simulink model "DDCU_wxt_v03"  (R2014a)
settings: Solver=ode45  StartTime=0.0  StopTime=50  FixedStep=0.0005  RelTol=1e-3
values from neighbouring files (symbols this model uses):
  ag_thr = 0.4*g    (= 3.924)    [Veh_Par_wxt.m]
  B = 2.25    [Veh_Par_wxt.m]
  bra_pre_em = 12    [Veh_Par_wxt.m]
  bra_pre_gz2 = 12/3    (= 4)    [Veh_Par_wxt.m]
  bra_pre_gz34 = 12/3    (= 4)    [Veh_Par_wxt.m]
  bra_pre_yd = 12/2    (= 6)    [Veh_Par_wxt.m]
  brakepre_dem_data = [0 1 2 3 4 5 6 7 8 9 10 11 12]    [Veh_Par_wxt.m]
  brakeTrq_dem_data = [0 218.198 436.396 654.594 872.792 1090.99 1309.188 1527.386 1745.584 1963.782 2181.98 2400.178 2618.376]    [Veh_Par_wxt.m]
  bratrq_max = 4*2618.376    (= 10473.504)    [Veh_Par_wxt.m]
  eff_tran = 0.75    [Veh_Par_wxt.m]
  G = Mass*g    (= 36297)    [Veh_Par_wxt.m]
  kd1 = 1    [Veh_Par_wxt.m]
  kd2 = 1    [Veh_Par_wxt.m]
  kd3 = 1    [Veh_Par_wxt.m]
  ki1 = 1    [Veh_Par_wxt.m]
  ki2 = 1    [Veh_Par_wxt.m]
  ki3 = 1    [Veh_Par_wxt.m]
  kp1 = 1    [Veh_Par_wxt.m]
  kp2 = 1    [Veh_Par_wxt.m]
  kp3 = 1    [Veh_Par_wxt.m]
  L = 3.12    [Veh_Par_wxt.m]
  premax = 12    [Veh_Par_wxt.m]
  Radius = 0.20    (= 0.2)    [Veh_Par_wxt.m]
  s_opt_yi_add = 0.05    [Veh_Par_wxt.m]
  s_opt_zhuan_add = 0.05    [Veh_Par_wxt.m]
  spd_map_mot = [0 100 200 300 360 400 500 600 700 800 900]*tras_ratio    [Veh_Par_wxt.m]
  spdmax = 900*tras_ratio    (= 5580)    [Veh_Par_wxt.m]
  speed_thr_park = 5/3.6/Radius*30/pi    (= 66.3145596216)    [Veh_Par_wxt.m]
  tras_ratio = 6.2    [Veh_Par_wxt.m]
  trq_map_mot = [1200 1200 1200 1200 1200 1080 864 720 617 540 480]/tras_ratio    [Veh_Par_wxt.m]
  trqmax = 80    [Veh_Par_wxt.m]
  v_thr1_b = 5    [Veh_Par_wxt.m]
  v_thr2_b = 20    [Veh_Par_wxt.m]
  v_thr_park = 5    [Veh_Par_wxt.m]
undefined symbols (not defined in the file or in its folder): DiscIntNeverNeededParam
libraries: simulink x34, Solver_SF x1
(part 4 of 10)

== system DDCU_wxt_v03/MainControl/mode_control/center_steer/center_steer/左右侧电机分配及功率限制 ==
  steer_dem : Inport
  pwr_dis_bat : Inport  Port=2
  speed_act_lf : Inport  Port=3
  speed_act_lr : Inport  Port=4
  speed_act_rf : Inport  Port=5
  speed_act_rr : Inport  Port=6
  TrqLimU_dig_lf : Inport  Port=7
  TrqLimU_dig_lr : Inport  Port=8
  TrqLimU_dig_rf : Inport  Port=9
  TrqLimU_dig_rr : Inport  Port=10
  Abs : Abs
  Add1 : Sum  Inputs=++++
  Add3 : Sum  Inputs=++++
  Constant : Constant  Value=9549
  Divide : Product  Inputs=**/
  Gain : Gain  Gain=1/4
  Gain1 : Gain  Gain=1/2
  Gain2 : Gain  Gain=1/100
  MinMax{,3..6} (5 alike) : MinMax  Inputs=2
  Product : Product
  mot_map{,1..3} (4 alike) : Lookup_n-D  NumberOfTableDimensions=1  BreakpointsForDimension1=spd_map_mot  Table=trq_map_mot  InternalRulePriority=Speed  RndMeth=Simplest  InputSameDT=on
  trq_dem_l : Outport
  trq_dem_r : Outport  Port=2
  trqlim_lf : Outport  Port=3
  trqlim_lr : Outport  Port=4
  trqlim_rf : Outport  Port=5
  trqlim_rr : Outport  Port=6
  wires:
  speed_act_rf/1 -> mot_map2/1, Add1/3
  speed_act_lr/1 -> mot_map1/1, Add1/2
  speed_act_rr/1 -> mot_map3/1, Add1/4
  speed_act_lf/1 -> mot_map/1, Add1/1
  Add1/1 -> Gain/1
  Constant/1 -> Divide/1
  pwr_dis_bat/1 -> Divide/2
  Gain/1 -> Divide/3
  mot_map3/1 -> MinMax3/1
  TrqLimU_dig_rr/1 -> MinMax3/2
  mot_map2/1 -> MinMax4/1
  TrqLimU_dig_rf/1 -> MinMax4/2
  mot_map1/1 -> MinMax5/1
  TrqLimU_dig_lr/1 -> MinMax5/2
  mot_map/1 -> MinMax6/1
  TrqLimU_dig_lf/1 -> MinMax6/2
  MinMax6/1 -> trqlim_lf/1, Add3/1
  MinMax5/1 -> trqlim_lr/1, Add3/2
  MinMax4/1 -> trqlim_rf/1, Add3/3
  MinMax3/1 -> trqlim_rr/1, Add3/4
  Divide/1 -> MinMax/1
  Add3/1 -> MinMax/2
  MinMax/1 -> Product/2
  steer_dem/1 -> Abs/1
  Product/1 -> Gain1/1
  Gain1/1 -> trq_dem_r/1, trq_dem_l/1
  Gain2/1 -> Product/1
  Abs/1 -> Gain2/1

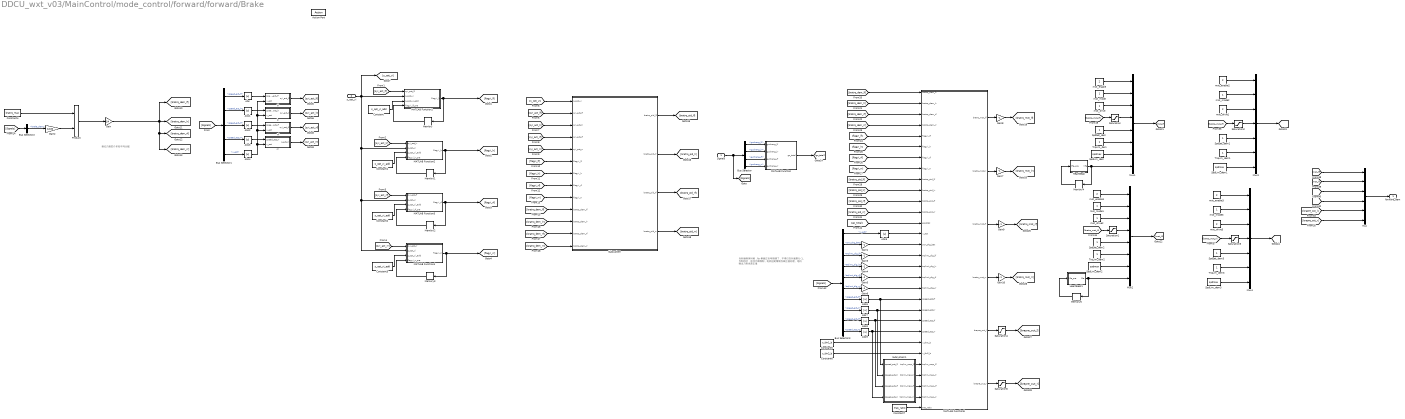
== system DDCU_wxt_v03/MainControl/mode_control/forward/forward/Brake ==
  note: 当时编程序时候，fcn里面正负号搞错了，不得已在外面乘以-1，
      | 当制动时，电池功率限制，电机扭矩限制当做正值处理，电机
      | 输出力矩也是正值
  note: 制动力矩四个车轮平均分配
  Signals : Inport
  s_opt_yi : Inport  Port=2
  Action Port : ActionPort
  Abs{,1..9} (10 alike) : Abs
  Bus Selector : BusSelector  OutputSignals=DriveMotor.guzhang_lf,DriveMotor.guzhang_lr,DriveMotor.guzhang_rf,DriveMotor.guzhang_rr
  Bus Selector1 : BusSelector  OutputSignals=DriveMotor.speed_act_lf,DriveMotor.speed_act_lr,DriveMotor.speed_act_rf,DriveMotor.speed_act_rr,IMU.v_act
  Bus Selector2 : BusSelector  OutputSignals=YaoKong.brake_dem
  Bus Selector3 : BusSelector  OutputSignals=IMU.v_act,Bat.pwr_chg_bat,DriveMotor.trqlimL_dig_lf,DriveMotor.trqlimL_dig_lr,DriveMotor.trqlimL_dig_rf,DriveMotor.trqlimL_dig_rr,DriveMotor.speed_act_lf,DriveMotor.speed_act_lr,DriveMotor.speed_act_rf,DriveMotor.speed_act_rr
  Constant{,1..3} (4 alike) : Constant  Value=s_opt_yi_add
  Constant4 : Constant  Value=bratrq_max
  Constant5 : Constant  Value=v_thr1_b
  Constant6 : Constant  Value=v_thr2_b
  Constant7 : Constant  Value=tras_ratio
  Gain : Gain  Gain=1/4
  Gain{1,3..10} (9 alike) : Gain  Gain=-1
  Gain2 : Gain  Gain=1/100
  HeartBeat : MATLAB Function  TreatAsAtomicUnit=on
  HeartBeat1 : MATLAB Function  TreatAsAtomicUnit=on
  MATLAB Function : MATLAB Function  TreatAsAtomicUnit=on
  MATLAB Function1 : MATLAB Function  TreatAsAtomicUnit=on
  MATLAB Function2 : MATLAB Function  TreatAsAtomicUnit=on
  MATLAB Function3 : MATLAB Function  TreatAsAtomicUnit=on
  MATLAB Function4 : MATLAB Function  TreatAsAtomicUnit=on
  MATLAB Function5 : MATLAB Function  TreatAsAtomicUnit=on
  Memory{,1..5} (6 alike) : Memory  InheritSampleTime=on
  Mux : Mux  Inputs=6
  Mux1 : Mux  Inputs=8
  Mux2 : Mux  Inputs=8
  Mux3 : Mux  Inputs=7
  Mux4 : Mux  Inputs=7
  Product : Product
  Saturation{,1..3} (4 alike) : Saturate  UpperLimit=0  LowerLimit=-trqmax
  Saturation4 : Saturate  UpperLimit=premax  LowerLimit=0
  Saturation5 : Saturate  UpperLimit=premax  LowerLimit=0
  SpdLim_dem{,1..3} (4 alike) : Constant  Value=spdmax
  SpdSet_dem{,1..3} (4 alike) : Constant
  Subsystem : Subsystem
  Subsystem1 : Subsystem
  TrqLim_dem{,1..3} (4 alike) : Constant
  lf : Subsystem
  lr : Subsystem
  mot_drive : Constant
  mot_drive1 : Constant  Value=2
  mot_drive2 : Constant
  mot_drive3 : Constant  Value=2
  mot_enable{,1..3} (4 alike) : Constant  Value=2
  mot_mode{,1..3} (4 alike) : Constant
  rf : Subsystem
  rr : Subsystem
  forward_dem : Outport
  wires:
  Signals/1 -> [Signals], Bus Selector/1
  Bus Selector/3 -> MATLAB Function/3(guzhang_rf)  "<guzhang_rf>"
  Bus Selector/4 -> MATLAB Function/4(guzhang_rr)  "<guzhang_rr>"
  Bus Selector/2 -> MATLAB Function/2(guzhang_lr)  "<guzhang_lr>"
  Bus Selector/1 -> MATLAB Function/1(guzhang_lf)  "<guzhang_lf>"
  MATLAB Function/1(gz_total) -> [gz_total]
  [Signals] -> Bus Selector1/1
  Bus Selector1/1 -> Abs/1  "<speed_act_lf>"
  Bus Selector1/2 -> Abs1/1  "<speed_act_lr>"
  Bus Selector1/3 -> Abs2/1  "<speed_act_rf>"
  Bus Selector1/4 -> Abs3/1  "<speed_act_rr>"
  Bus Selector1/5 -> Abs4/1  "<v_act>"
  Constant3/1 -> MATLAB Function4/3(s_opt_yi_add)
  Memory3/1 -> MATLAB Function4/4(flagyi_rr_pre)
  MATLAB Function4/1(flagyi_rr) -> Memory3/1, [flagyi_rr]
  s_opt_yi/1 -> MATLAB Function2/2(s_opt_yi), MATLAB Function3/2(s_opt_yi), MATLAB Function4/2(s_opt_yi), MATLAB Function1/2(s_opt_yi), [s_opt_yi]
  Constant2/1 -> MATLAB Function3/3(s_opt_yi_add)
  Memory2/1 -> MATLAB Function3/4(flagyi_rf_pre)
  MATLAB Function3/1(flagyi_rf) -> [flagyi_rf], Memory2/1
  Constant1/1 -> MATLAB Function2/3(s_opt_yi_add)
  Memory1/1 -> MATLAB Function2/4(flagyi_lr_pre)
  MATLAB Function2/1(flagyi_lr) -> Memory1/1, [flagyi_lr]
  Constant/1 -> MATLAB Function1/3(s_opt_yi_add)
  Memory/1 -> MATLAB Function1/4(flagyi_lf_pre)
  MATLAB Function1/1(flagyi_lf) -> [flagyi_lf], Memory/1
  lr/1(syi_act_lr) -> [syi_act_lr]
  lf/1(syi_act_lf) -> [syi_act_lf]
  rf/1(syi_act_rf) -> [syi_act_rf]
  rr/1(s_act_rr) -> [syi_act_rr]
  [syi_act_lf] -> MATLAB Function1/1(syi_act_lf)
  [syi_act_lr] -> MATLAB Function2/1(syi_act_lr)
  [syi_act_rf] -> MATLAB Function3/1(syi_act_rf)
  [syi_act_rr] -> MATLAB Function4/1(syi_act_rr)
  [s_opt_yi] -> Subsystem/1(s_opt_yi)
  [syi_act_lf] -> Subsystem/2(syi_act_lf)
  [syi_act_lr] -> Subsystem/3(syi_act_lr)
  [syi_act_rf] -> Subsystem/4(syi_act_rf)
  [syi_act_rr] -> Subsystem/5(syi_act_rr)
  [flagyi_rf] -> Subsystem/8(flagyi_rf)
  [flagyi_lf] -> Subsystem/6(flagyi_lf)
  [flagyi_lr] -> Subsystem/7(flagyi_lr)
  [flagyi_rr] -> Subsystem/9(flagyi_rr)
  [Signals] -> Bus Selector2/1
  Gain/1 -> [bratrq_dem_lr], [bratrq_dem_rr], [bratrq_dem_rf], [bratrq_dem_lf]
  [bratrq_dem_lf] -> Subsystem/10(bratrq_dem_lf)
  [bratrq_dem_lr] -> Subsystem/11(bratrq_dem_lr)
  [bratrq_dem_rf] -> Subsystem/12(bratrq_dem_rf)
  [bratrq_dem_rr] -> Subsystem/13(bratrq_dem_rr)
  Subsystem/2(bratrq_pid_lr) -> [bratrq_pid_lr]
  Subsystem/3(bratrq_pid_rf) -> [bratrq_pid_rf]
  Subsystem/1(bratrq_pid_lf) -> [bratrq_pid_lf]
  Subsystem/4(bratrq_pid_rr) -> [bratrq_pid_rr]
  Mux/1 -> forward_dem/1
  SpdLim_dem3/1 -> Mux4/7
  TrqLim_dem3/1 -> Mux4/6
  Mux4/1 -> [mot_rr]
  SpdSet_dem3/1 -> Mux4/5
  mot_enable3/1 -> Mux4/1
  [bratrq_mot_rr] -> Saturation3/1
  mot_mode3/1 -> Mux4/2
  mot_drive3/1 -> Mux4/3
  SpdLim_dem2/1 -> Mux2/7
  Memory5/1 -> HeartBeat1/1(life_pre)
  HeartBeat1/1(life) -> Memory5/1, Mux2/8
  TrqLim_dem2/1 -> Mux2/6
  Mux2/1 -> [mot_lr]
  SpdSet_dem2/1 -> Mux2/5
  mot_enable1/1 -> Mux2/1
  [bratrq_mot_lr] -> Saturation1/1
  mot_mode1/1 -> Mux2/2
  mot_drive2/1 -> Mux2/3
  SpdLim_dem1/1 -> Mux3/7
  TrqLim_dem1/1 -> Mux3/6
  Mux3/1 -> [mot_rf]
  SpdSet_dem1/1 -> Mux3/5
  mot_enable2/1 -> Mux3/1
  [bratrq_mot_rf] -> Saturation2/1
  mot_mode2/1 -> Mux3/2
  mot_drive1/1 -> Mux3/3
  SpdLim_dem/1 -> Mux1/7
  Memory4/1 -> HeartBeat/1(life_pre)
  HeartBeat/1(life) -> Memory4/1, Mux1/8
  TrqLim_dem/1 -> Mux1/6
  Mux1/1 -> [mot_lf]
  SpdSet_dem/1 -> Mux1/5
  mot_enable/1 -> Mux1/1
  mot_mode/1 -> Mux1/2
  mot_drive/1 -> Mux1/3
  [mot_lf] -> Mux/1
  [mot_lr] -> Mux/2
  [mot_rf] -> Mux/3
  [mot_rr] -> Mux/4
  [brapre_out_l] -> Mux/5
  [brapre_out_r] -> Mux/6
  MATLAB Function5/1(bratrq_mot_lf) -> Gain8/1
  MATLAB Function5/3(bratrq_mot_rf) -> Gain9/1
  MATLAB Function5/2(bratrq_mot_lr) -> Gain7/1
  MATLAB Function5/4(bratrq_mot_rr) -> Gain10/1
  MATLAB Function5/5(brapre_out_l) -> Saturation4/1
  MATLAB Function5/6(brapre_out_r) -> Saturation5/1
  [Signals] -> Bus Selector3/1
  Bus Selector3/2 -> Gain1/1  "<pwr_chg_bat>"
  Bus Selector3/1 -> Abs5/1  "<v_act>"
  Bus Selector3/3 -> Gain3/1  "<trqlimL_dig_lf>"
  Bus Selector3/4 -> Gain4/1  "<trqlimL_dig_lr>"
  Bus Selector3/5 -> Gain5/1  "<trqlimL_dig_rf>"
  Bus Selector3/6 -> Gain6/1  "<trqlimL_dig_rr>"
  Bus Selector3/7 -> Abs6/1  "<speed_act_lf>"
  Bus Selector3/8 -> Abs7/1  "<speed_act_lr>"
  Bus Selector3/9 -> Abs8/1  "<speed_act_rf>"
  Bus Selector3/10 -> Abs9/1  "<speed_act_rr>"
  Constant4/1 -> Product/1
  Gain2/1 -> Product/2
  Bus Selector2/1 -> Gain2/1  "<brake_dem>"
  Product/1 -> Gain/1
  Constant6/1 -> MATLAB Function5/25(v_thr2_b)
  Gain1/1 -> MATLAB Function5/15(pwr_chg_bat)
  Gain3/1 -> MATLAB Function5/16(trqlimL_dig_lf)
  Gain4/1 -> MATLAB Function5/17(trqlimL_dig_lr)
  Gain5/1 -> MATLAB Function5/18(trqlimL_dig_rf)
  Gain6/1 -> MATLAB Function5/19(trqlimL_dig_rr)
  [bratrq_dem_lr] -> MATLAB Function5/2(bratrq_dem_lr)
  [bratrq_dem_rf] -> MATLAB Function5/3(bratrq_dem_rf)
  [bratrq_dem_lf] -> MATLAB Function5/1(bratrq_dem_lf)
  [bratrq_dem_rr] -> MATLAB Function5/4(bratrq_dem_rr)
  [flagyi_lf] -> MATLAB Function5/5(flagyi_lf)
  [flagyi_lr] -> MATLAB Function5/6(flagyi_lr)
  [flagyi_rf] -> MATLAB Function5/7(flagyi_rf)
  [flagyi_rr] -> MATLAB Function5/8(flagyi_rr)
  [bratrq_pid_lf] -> MATLAB Function5/9(bratrq_pid_lf)
  [bratrq_pid_lr] -> MATLAB Function5/10(bratrq_pid_lr)
  [bratrq_pid_rf] -> MATLAB Function5/11(bratrq_pid_rf)
  [bratrq_pid_rr] -> MATLAB Function5/12(bratrq_pid_rr)
  [gz_total] -> MATLAB Function5/13(gz_total)
  Subsystem1/4(trqlim_map_rr) -> MATLAB Function5/29(trqlim_map_rr)
  Subsystem1/3(trqlim_map_rf) -> MATLAB Function5/28(trqlim_map_rf)
  Subsystem1/2(trqlim_map_lr) -> MATLAB Function5/27(trqlim_map_lr)
  Subsystem1/1(trqlim_map_lf) -> MATLAB Function5/26(trqlim_map_lf)
  Constant5/1 -> MATLAB Function5/24(v_thr1_b)
  [bratrq_mot_lf] -> Saturation/1
  Gain8/1 -> [bratrq_mot_lf]
  Gain7/1 -> [bratrq_mot_lr]
  Gain9/1 -> [bratrq_mot_rf]
  Gain10/1 -> [bratrq_mot_rr]
  Saturation/1 -> Mux1/4
  Saturation1/1 -> Mux2/4
  Saturation2/1 -> Mux3/4
  Saturation3/1 -> Mux4/4
  Saturation4/1 -> [brapre_out_l]
  Saturation5/1 -> [brapre_out_r]
  Abs/1 -> lf/1(speed_act_lf)
  Abs1/1 -> lr/1(speed_act_lr)
  Abs2/1 -> rf/1(speed_act_rf)
  Abs3/1 -> rr/1(speed_act_rr)
  Abs4/1 -> rr/2(v_act), rf/2(v_act), lr/2(v_act), lf/2(v_act)
  Abs5/1 -> MATLAB Function5/14(v_act)
  Abs6/1 -> Subsystem1/1(speed_act_lf), MATLAB Function5/20(speed_act_lf)
  Abs7/1 -> Subsystem1/2(speed_act_lr), MATLAB Function5/21(speed_act_lr)
  Abs8/1 -> Subsystem1/3(speed_act_rf), MATLAB Function5/22(speed_act_rf)
  Abs9/1 -> Subsystem1/4(speed_act_rr), MATLAB Function5/23(speed_act_rr)
  Constant7/1 -> MATLAB Function5/30(tras_ratio)

== system DDCU_wxt_v03/MainControl/mode_control/forward/forward/Drive ==
  Signals : Inport
  Action Port : ActionPort
  Abs{,1..10} (11 alike) : Abs
  Bus Selector : BusSelector  OutputSignals=YaoKong.acc_dem,IMU.v_act,DriveMotor.trqlimU_dig_lf,DriveMotor.trqlimU_dig_lr,DriveMotor.trqlimU_dig_rf,DriveMotor.trqlimU_dig_rr
  Bus Selector1 : BusSelector  OutputSignals=IMU.acc_y
  Bus Selector2 : BusSelector  OutputSignals=IMU.acc_y,YaoKong.steer_dem
  Bus Selector3 : BusSelector  OutputSignals=IMU.dis_east,IMU.dis_north,IMU.hangxiangangle
  Bus Selector4 : BusSelector  OutputSignals=IMU.v_act,DriveMotor.trqlimU_dig_lf,DriveMotor.trqlimU_dig_lr,DriveMotor.trqlimU_dig_rf,DriveMotor.trqlimU_dig_rr,YaoKong.steer_dem
  Bus Selector5 : BusSelector  OutputSignals=Bat.pwr_dis_bat,DriveMotor.speed_act_lf,DriveMotor.speed_act_lr,DriveMotor.speed_act_rf,DriveMotor.speed_act_rr,DriveMotor.trqlimU_dig_lf,DriveMotor.trqlimU_dig_lr,DriveMotor.trqlimU_dig_rf,DriveMotor.trqlimU_dig_rr
  Bus Selector6 : BusSelector  OutputSignals=DriveMotor.guzhang_lf,DriveMotor.guzhang_lr,DriveMotor.guzhang_rf,DriveMotor.guzhang_rr
  Bus Selector7 : BusSelector  OutputSignals=DriveMotor.speed_act_lf,DriveMotor.speed_act_lr,DriveMotor.speed_act_rf,DriveMotor.speed_act_rr,IMU.v_act,YaoKong.steer_dem,IMU.acc_y,YaoKong.brake_dem
  Constant : Constant  Value=ag_thr
  Constant1 : Constant
  MATLAB Function : MATLAB Function  TreatAsAtomicUnit=on
  Multiport Switch : MultiPortSwitch  DataPortOrder=Zero-based contiguous
  Scope : Scope
      settings: SaveName=ScopeData5
  Scope1 : Scope
      settings: SaveName=ScopeData6
  Scope2 : Scope
      settings: SaveName=ScopeData9
  Switch Case : SwitchCase  CaseConditions={0,1,2}  ShowDefaultCase=off
  Terminator : Terminator
  容错控制 : Subsystem
  左右侧电机分配及功率限制 : Subsystem
  目标直驶力矩确定模块 : Subsystem
  目标转向力矩确定模块 : Subsystem  TreatAsAtomicUnit=on
  直驶纠偏控制 : Subsystem  TreatAsAtomicUnit=on
  路面状况识别模块 : Subsystem
  车辆稳定性控制 : Subsystem  TreatAsAtomicUnit=on
  驱动防滑控制TCS : Subsystem
  forward_dem : Outport
  wires:
  Signals/1 -> [Signals], Bus Selector4/1, Bus Selector3/1, Bus Selector1/1, Bus Selector2/1, Bus Selector/1
  Bus Selector/1 -> 目标直驶力矩确定模块/1(acc_dem)  "<acc_dem>"
  Bus Selector/2 -> Abs9/1  "<v_act>"
  Bus Selector1/1 -> 车辆稳定性控制/1(acc_y)  "<acc_y>"
  MATLAB Function/1(y) -> Scope2/1, Multiport Switch/1, Switch Case/1
  Switch Case/1 -> 车辆稳定性控制/Action
  Switch Case/2 -> 目标转向力矩确定模块/Action
  Switch Case/3 -> 直驶纠偏控制/Action
  车辆稳定性控制/1(delta_Twending_dem) -> Multiport Switch/2
  目标转向力矩确定模块/1(delta_Tsteer_dem) -> Scope/1, Multiport Switch/3
  直驶纠偏控制/1(delta_Tjiupian) -> Multiport Switch/4
  Bus Selector2/2 -> MATLAB Function/2(steer_dem)  "<steer_dem>"
  Constant/1 -> MATLAB Function/3(ag_thr)
  [umax] -> 目标转向力矩确定模块/7(umax)
  [f] -> 目标转向力矩确定模块/8(f)
  路面状况识别模块/1(umax) -> [umax]
  路面状况识别模块/2(f) -> [f]
  路面状况识别模块/3(s_opt_zhuan) -> [s_opt_zhuan]
  Bus Selector3/1 -> 直驶纠偏控制/1(dis_east)  "<dis_east>"
  Bus Selector3/2 -> 直驶纠偏控制/2(dis_north)  "<dis_north>"
  Bus Selector3/3 -> 直驶纠偏控制/3(hangxiangangle)  "<hangxiangangle>"
  Multiport Switch/1 -> Scope1/1, 左右侧电机分配及功率限制/2(delta_T_dem)
  目标直驶力矩确定模块/1(Trq_line_dem) -> 左右侧电机分配及功率限制/1(Trq_line_dem)
  Bus Selector/4 -> 目标直驶力矩确定模块/4(TrqLimU_dig_lr)  "<trqlimU_dig_lr>"
  Bus Selector/3 -> 目标直驶力矩确定模块/3(TrqLimU_dig_lf)  "<trqlimU_dig_lf>"
  Bus Selector/5 -> 目标直驶力矩确定模块/5(TrqLimU_dig_rf)  "<trqlimU_dig_rf>"
  Bus Selector/6 -> 目标直驶力矩确定模块/6(TrqLimU_dig_rr)  "<trqlimU_dig_rr>"
  Bus Selector4/4 -> 目标转向力矩确定模块/4(TrqLimU_dig_rf)  "<trqlimU_dig_rf>"
  Bus Selector4/5 -> 目标转向力矩确定模块/5(TrqLimU_dig_rr)  "<trqlimU_dig_rr>"
  Bus Selector4/6 -> 目标转向力矩确定模块/6(steer_dem)  "<steer_dem>"
  Bus Selector4/1 -> Abs10/1  "<v_act>"
  Bus Selector4/2 -> 目标转向力矩确定模块/2(TrqLimU_dig_lf)  "<trqlimU_dig_lf>"
  Bus Selector4/3 -> 目标转向力矩确定模块/3(TrqLimU_dig_lr)  "<trqlimU_dig_lr>"
  Bus Selector2/1 -> MATLAB Function/1(acc_y)  "<acc_y>"
  [Signals] -> Bus Selector5/1
  Bus Selector5/1 -> 左右侧电机分配及功率限制/3(pwr_dis_bat)  "<pwr_dis_bat>"
  Bus Selector5/2 -> Abs/1  "<speed_act_lf>"
  Bus Selector5/3 -> Abs1/1  "<speed_act_lr>"
  Bus Selector5/4 -> Abs2/1  "<speed_act_rf>"
  Bus Selector5/5 -> Abs3/1  "<speed_act_rr>"
  Bus Selector5/9 -> 左右侧电机分配及功率限制/11(TrqLimU_dig_rr)  "<trqlimU_dig_rr>"
  Bus Selector5/8 -> 左右侧电机分配及功率限制/10(TrqLimU_dig_rf)  "<trqlimU_dig_rf>"
  Bus Selector5/6 -> 左右侧电机分配及功率限制/8(TrqLimU_dig_lf)  "<trqlimU_dig_lf>"
  Bus Selector5/7 -> 左右侧电机分配及功率限制/9(TrqLimU_dig_lr)  "<trqlimU_dig_lr>"
  [Signals] -> Bus Selector6/1
  左右侧电机分配及功率限制/2(trq_dem_r) -> 容错控制/2(trq_dem_r)
  左右侧电机分配及功率限制/1(trq_dem_l) -> 容错控制/1(trq_dem_l)
  Bus Selector6/4 -> 容错控制/10(guzhang_rr)  "<guzhang_rr>"
  Bus Selector6/3 -> 容错控制/9(guzhang_rf)  "<guzhang_rf>"
  Bus Selector6/2 -> 容错控制/8(guzhang_lr)  "<guzhang_lr>"
  Bus Selector6/1 -> 容错控制/7(guzhang_lf)  "<guzhang_lf>"
  左右侧电机分配及功率限制/5(trqlim_rf) -> 容错控制/5(trqlim_rf)
  左右侧电机分配及功率限制/4(trqlim_lr) -> 容错控制/4(trqlim_lr)
  左右侧电机分配及功率限制/6(trqlim_rr) -> 容错控制/6(trqlim_rr)
  左右侧电机分配及功率限制/3(trqlim_lf) -> 容错控制/3(trqlim_lf)
  容错控制/1(trq_dem_lf) -> 驱动防滑控制TCS/1(trq_dem_lf)
  容错控制/5(bra_pre_l) -> 驱动防滑控制TCS/5(bra_pre_l)
  容错控制/6(bra_pre_r) -> 驱动防滑控制TCS/6(bra_pre_r)
  容错控制/2(trq_dem_lr) -> 驱动防滑控制TCS/2(trq_dem_lr)
  容错控制/3(trq_dem_rf) -> 驱动防滑控制TCS/3(trq_dem_rf)
  容错控制/4(trq_dem_rr) -> 驱动防滑控制TCS/4(trq_dem_rr)
  Bus Selector7/7 -> 驱动防滑控制TCS/13(acc_y)  "<acc_y>"
  Bus Selector7/6 -> 驱动防滑控制TCS/12(steer_dem)  "<steer_dem>"
  Bus Selector7/5 -> Abs8/1  "<v_act>"
  Bus Selector7/4 -> Abs7/1  "<speed_act_rr>"
  Bus Selector7/3 -> Abs6/1  "<speed_act_rf>"
  Bus Selector7/2 -> Abs5/1  "<speed_act_lr>"
  Bus Selector7/1 -> Abs4/1  "<speed_act_lf>"
  [s_opt_zhuan] -> 驱动防滑控制TCS/15(s_opt_zhuan)
  Bus Selector7/8 -> 驱动防滑控制TCS/14(brake_dem)  "<brake_dem>"
  [Signals] -> Bus Selector7/1
  驱动防滑控制TCS/1(forward_dem) -> forward_dem/1
  Constant1/1 -> 路面状况识别模块/1(In1)
  路面状况识别模块/4(s_opt_yi) -> Terminator/1
  Abs/1 -> 左右侧电机分配及功率限制/4(speed_act_lf)
  Abs1/1 -> 左右侧电机分配及功率限制/5(speed_act_lr)
  Abs2/1 -> 左右侧电机分配及功率限制/6(speed_act_rf)
  Abs3/1 -> 左右侧电机分配及功率限制/7(speed_act_rr)
  Abs4/1 -> 驱动防滑控制TCS/7(speed_act_lf)
  Abs5/1 -> 驱动防滑控制TCS/8(speed_act_lr)
  Abs6/1 -> 驱动防滑控制TCS/9(speed_act_rf)
  Abs7/1 -> 驱动防滑控制TCS/10(speed_act_rr)
  Abs8/1 -> 驱动防滑控制TCS/11(v_act)
  Abs9/1 -> 目标直驶力矩确定模块/2(v_act)
  Abs10/1 -> 目标转向力矩确定模块/1(v_act)

== system DDCU_wxt_v03/MainControl/mode_control/backward/backward/Brake/Subsystem ==
  s_opt_yi : Inport
  syi_act_lf : Inport  Port=2
  syi_act_lr : Inport  Port=3
  syi_act_rf : Inport  Port=4
  syi_act_rr : Inport  Port=5
  flagyi_lf : Inport  Port=6
  flagyi_lr : Inport  Port=7
  flagyi_rf : Inport  Port=8
  flagyi_rr : Inport  Port=9
  bratrq_dem_lf : Inport  Port=10
  bratrq_dem_lr : Inport  Port=11
  bratrq_dem_rf : Inport  Port=12
  bratrq_dem_rr : Inport  Port=13
  Add{1..2,5,7} (4 alike) : Sum  Inputs=+++
  Add{3..4,6,8} (4 alike) : Sum
  Difference{,1..3} (4 alike) : simulink/Discrete/Difference  ICPrevInput=0.0  InputProcessing=Inherited  OutMin=[]  OutMax=[]  OutDataType=fixdt(1, 16)  OutScaling=2^-10  DoSatur=off
  Discrete-Time Integrator{,1..3} (4 alike) : DiscreteIntegrator  SampleTime=-1  ICPrevOutput=DiscIntNeverNeededParam  ICPrevScaledInput=DiscIntNeverNeededParam
  Gain{1,4,7,10} (4 alike) : Gain  Gain=kp3
  Gain{2,5,8,11} (4 alike) : Gain  Gain=ki3
  Gain{3,6,9,12} (4 alike) : Gain  Gain=kd3
  Sum{,1..3} (4 alike) : Sum  Inputs=|+-
  Switch{,1..3} (4 alike) : Switch  Criteria=u2 > Threshold  Threshold=0.5
  bratrq_pid_lf : Outport
  bratrq_pid_lr : Outport  Port=2
  bratrq_pid_rf : Outport  Port=3
  bratrq_pid_rr : Outport  Port=4
  wires:
  Sum2/1 -> Gain7/1, Gain9/1, Gain8/1
  Add5/1 -> Add6/1
  Sum3/1 -> Gain10/1, Gain12/1, Gain11/1
  Add7/1 -> Add8/1
  Sum1/1 -> Gain4/1, Gain5/1, Gain6/1
  Sum/1 -> Gain1/1, Gain3/1, Gain2/1
  Switch3/1 -> bratrq_pid_rf/1
  flagyi_rf/1 -> Switch3/2
  [s_opt_yi] -> Sum3/1
  Gain11/1 -> Discrete-Time Integrator3/1
  Gain10/1 -> Add7/1
  Gain12/1 -> Difference3/1
  Discrete-Time Integrator3/1 -> Add7/2
  Difference3/1 -> Add7/3
  syi_act_rf/1 -> Sum3/2
  bratrq_dem_rf/1 -> Add8/2, Switch3/3
  Add8/1 -> Switch3/1
  Switch2/1 -> bratrq_pid_rr/1
  flagyi_rr/1 -> Switch2/2
  [s_opt_yi] -> Sum2/1
  Gain8/1 -> Discrete-Time Integrator2/1
  Gain7/1 -> Add5/1
  Gain9/1 -> Difference2/1
  Discrete-Time Integrator2/1 -> Add5/2
  Difference2/1 -> Add5/3
  syi_act_rr/1 -> Sum2/2
  bratrq_dem_rr/1 -> Add6/2, Switch2/3
  Add6/1 -> Switch2/1
  Switch1/1 -> bratrq_pid_lr/1
  flagyi_lr/1 -> Switch1/2
  [s_opt_yi] -> Sum1/1
  Gain5/1 -> Discrete-Time Integrator1/1
  Gain4/1 -> Add1/1
  Gain6/1 -> Difference1/1
  Discrete-Time Integrator1/1 -> Add1/2
  Difference1/1 -> Add1/3
  syi_act_lr/1 -> Sum1/2
  bratrq_dem_lr/1 -> Add4/2, Switch1/3
  Add4/1 -> Switch1/1
  Switch/1 -> bratrq_pid_lf/1
  flagyi_lf/1 -> Switch/2
  s_opt_yi/1 -> Sum/1, [s_opt_yi]
  Gain2/1 -> Discrete-Time Integrator/1
  Gain1/1 -> Add2/1
  Gain3/1 -> Difference/1
  Discrete-Time Integrator/1 -> Add2/2
  Difference/1 -> Add2/3
  syi_act_lf/1 -> Sum/2
  bratrq_dem_lf/1 -> Add3/2, Switch/3
  Add3/1 -> Switch/1
  Add2/1 -> Add3/1
  Add1/1 -> Add4/1

== system DDCU_wxt_v03/MainControl/mode_control/backward/backward/Brake/Subsystem1 ==
  speed_act_lf : Inport
  speed_act_lr : Inport  Port=2
  speed_act_rf : Inport  Port=3
  speed_act_rr : Inport  Port=4
  mot_map{,1..3} (4 alike) : Lookup_n-D  NumberOfTableDimensions=1  BreakpointsForDimension1=spd_map_mot  Table=trq_map_mot  InternalRulePriority=Speed  RndMeth=Simplest  InputSameDT=on
  trqlim_map_lf : Outport
  trqlim_map_lr : Outport  Port=2
  trqlim_map_rf : Outport  Port=3
  trqlim_map_rr : Outport  Port=4
  wires:
  mot_map3/1 -> trqlim_map_rr/1
  mot_map2/1 -> trqlim_map_rf/1
  mot_map1/1 -> trqlim_map_lr/1
  mot_map/1 -> trqlim_map_lf/1
  speed_act_rr/1 -> mot_map3/1
  speed_act_rf/1 -> mot_map2/1
  speed_act_lr/1 -> mot_map1/1
  speed_act_lf/1 -> mot_map/1

== system DDCU_wxt_v03/MainControl/mode_control/backward/backward/Brake/lf ==
  speed_act_lf : Inport
  v_act : Inport  Port=2
  Add : Sum
  Constant : Constant  Value=eps
  Divide : Product  Inputs=*/
  Gain : Gain  Gain=pi/30
  Gain1 : Gain  Gain=Radius
  Gain2 : Gain  Gain=1/3.6
  Subtract : Sum  Inputs=+-
  syi_act_lf : Outport
  wires:
  Gain1/1 -> Subtract/2
  Gain2/1 -> Subtract/1, Add/1
  speed_act_lf/1 -> Gain/1
  Gain/1 -> Gain1/1
  v_act/1 -> Gain2/1
  Subtract/1 -> Divide/1
  Constant/1 -> Add/2
  Add/1 -> Divide/2
  Divide/1 -> syi_act_lf/1

== system DDCU_wxt_v03/MainControl/mode_control/backward/backward/Brake/lr ==
  speed_act_lr : Inport
  v_act : Inport  Port=2
  Add : Sum
  Constant : Constant  Value=eps
  Divide : Product  Inputs=*/
  Gain : Gain  Gain=pi/30
  Gain1 : Gain  Gain=Radius
  Gain2 : Gain  Gain=1/3.6
  Subtract : Sum  Inputs=+-
  syi_act_lr : Outport
  wires:
  Gain2/1 -> Subtract/1, Add/1
  Gain1/1 -> Subtract/2
  Divide/1 -> syi_act_lr/1
  Add/1 -> Divide/2
  Constant/1 -> Add/2
  Subtract/1 -> Divide/1
  v_act/1 -> Gain2/1
  Gain/1 -> Gain1/1
  speed_act_lr/1 -> Gain/1

== system DDCU_wxt_v03/MainControl/mode_control/backward/backward/Brake/rf ==
  speed_act_rf : Inport
  v_act : Inport  Port=2
  Add : Sum
  Constant : Constant  Value=eps
  Divide : Product  Inputs=*/
  Gain : Gain  Gain=pi/30
  Gain1 : Gain  Gain=Radius
  Gain2 : Gain  Gain=1/3.6
  Subtract : Sum  Inputs=+-
  syi_act_rf : Outport
  wires:
  Gain1/1 -> Subtract/2
  Gain2/1 -> Subtract/1, Add/1
  speed_act_rf/1 -> Gain/1
  Gain/1 -> Gain1/1
  v_act/1 -> Gain2/1
  Subtract/1 -> Divide/1
  Constant/1 -> Add/2
  Add/1 -> Divide/2
  Divide/1 -> syi_act_rf/1

== system DDCU_wxt_v03/MainControl/mode_control/backward/backward/Brake/rr ==
  speed_act_rr : Inport
  v_act : Inport  Port=2
  Add : Sum
  Constant : Constant  Value=eps
  Divide : Product  Inputs=*/
  Gain : Gain  Gain=pi/30
  Gain1 : Gain  Gain=Radius
  Gain2 : Gain  Gain=1/3.6
  Subtract : Sum  Inputs=+-
  s_act_rr : Outport
  wires:
  Gain1/1 -> Subtract/2
  Gain2/1 -> Subtract/1, Add/1
  Divide/1 -> s_act_rr/1
  Add/1 -> Divide/2
  Constant/1 -> Add/2
  Subtract/1 -> Divide/1
  v_act/1 -> Gain2/1
  Gain/1 -> Gain1/1
  speed_act_rr/1 -> Gain/1

== system DDCU_wxt_v03/MainControl/mode_control/backward/backward/Drive/容错控制 ==
  trq_dem_l : Inport
  trq_dem_r : Inport  Port=2
  trqlim_lf : Inport  Port=3
  trqlim_lr : Inport  Port=4
  trqlim_rf : Inport  Port=5
  trqlim_rr : Inport  Port=6
  guzhang_lf : Inport  Port=7
  guzhang_lr : Inport  Port=8
  guzhang_rf : Inport  Port=9
  guzhang_rr : Inport  Port=10
  Add : Sum
  Add1 : Sum
  Constant : Constant  Value=bra_pre_gz2
  Constant1 : Constant  Value=bra_pre_gz34
  MATLAB Function : MATLAB Function  TreatAsAtomicUnit=on
  Mux : Mux  Inputs=2
  Scope{,1..16} (17 alike) : Scope
      Scope settings: SaveName=ScopeData25
      Scope1 settings: SaveName=ScopeData26
      Scope10 settings: SaveName=ScopeData35
      Scope11 settings: SaveName=ScopeData36
      Scope12 settings: SaveName=ScopeData37
      Scope13 settings: SaveName=ScopeData38
      Scope14 settings: SaveName=ScopeData39
      Scope15 settings: SaveName=ScopeData40
      Scope16 settings: SaveName=ScopeData41
      Scope2 settings: SaveName=ScopeData27
      Scope3 settings: SaveName=ScopeData28
      Scope4 settings: SaveName=ScopeData29
      Scope5 settings: SaveName=ScopeData30
      Scope6 settings: SaveName=ScopeData31
      Scope7 settings: SaveName=ScopeData32
      Scope8 settings: SaveName=ScopeData33
      Scope9 settings: SaveName=ScopeData34
  Subtract : Sum  Inputs=+-
  trq_dem_lf : Outport
  trq_dem_lr : Outport  Port=2
  trq_dem_rf : Outport  Port=3
  trq_dem_rr : Outport  Port=4
  bra_pre_l : Outport  Port=5
  bra_pre_r : Outport  Port=6
  wires:
  MATLAB Function/7(mode) -> Scope11/1
  Mux/1 -> Scope7/1
  Subtract/1 -> Scope6/1
  Add1/1 -> Subtract/2, Mux/2
  Add/1 -> Subtract/1, Mux/1
  Constant1/1 -> MATLAB Function/12(bra_pre_gz34)
  Constant/1 -> MATLAB Function/11(bra_pre_gz2)
  MATLAB Function/6(bra_pre_r) -> bra_pre_r/1, Scope5/1
  MATLAB Function/5(bra_pre_l) -> bra_pre_l/1, Scope4/1
  MATLAB Function/4(trq_dem_rr) -> trq_dem_rr/1, Add1/2, Scope3/1
  MATLAB Function/3(trq_dem_rf) -> trq_dem_rf/1, Add1/1, Scope2/1
  MATLAB Function/2(trq_dem_lr) -> trq_dem_lr/1, Add/2, Scope1/1
  MATLAB Function/1(trq_dem_lf) -> trq_dem_lf/1, Add/1, Scope/1
  trqlim_lf/1 -> MATLAB Function/3(trqlim_lf)
  trqlim_rr/1 -> MATLAB Function/6(trqlim_rr), Scope12/1
  trqlim_rf/1 -> MATLAB Function/5(trqlim_rf), Scope10/1
  trq_dem_l/1 -> MATLAB Function/1(trq_dem_l), Scope8/1
  trqlim_lr/1 -> MATLAB Function/4(trqlim_lr)
  trq_dem_r/1 -> MATLAB Function/2(trq_dem_r), Scope9/1
  guzhang_lf/1 -> MATLAB Function/7(guzhang_lf), Scope13/1
  guzhang_rr/1 -> MATLAB Function/10(guzhang_rr), Scope16/1
  guzhang_rf/1 -> MATLAB Function/9(guzhang_rf), Scope15/1
  guzhang_lr/1 -> Scope14/1, MATLAB Function/8(guzhang_lr)

== system DDCU_wxt_v03/MainControl/mode_control/backward/backward/Drive/左右侧电机分配及功率限制 ==
  Trq_line_dem : Inport
  delta_T_dem : Inport  Port=2
  pwr_dis_bat : Inport  Port=3
  speed_act_lf : Inport  Port=4
  speed_act_lr : Inport  Port=5
  speed_act_rf : Inport  Port=6
  speed_act_rr : Inport  Port=7
  TrqLimU_dig_lf : Inport  Port=8
  TrqLimU_dig_lr : Inport  Port=9
  TrqLimU_dig_rf : Inport  Port=10
  TrqLimU_dig_rr : Inport  Port=11
  Add : Sum
  Add1 : Sum  Inputs=++++
  Add2 : Sum
  Add3 : Sum
  Constant : Constant  Value=9549
  Divide : Product  Inputs=**/
  Gain : Gain  Gain=1/4
  Gain1 : Gain  Gain=1/2
  Gain2 : Gain  Gain=1/2
  MATLAB Function : MATLAB Function  TreatAsAtomicUnit=on
  MinMax{,1..6} (7 alike) : MinMax  Inputs=2
  Mux : Mux  Inputs=2
  Scope{,1..10} (11 alike) : Scope
      Scope settings: SaveName=ScopeData14
      Scope1 settings: SaveName=ScopeData15
      Scope10 settings: SaveName=ScopeData24
      Scope2 settings: SaveName=ScopeData16
      Scope3 settings: SaveName=ScopeData17
      Scope4 settings: SaveName=ScopeData18
      Scope5 settings: SaveName=ScopeData19
      Scope6 settings: SaveName=ScopeData20
      Scope7 settings: SaveName=ScopeData21
      Scope8 settings: SaveName=ScopeData22
      Scope9 settings: SaveName=ScopeData23
  Subtract : Sum  Inputs=+-
  mot_map{,1..3} (4 alike) : Lookup_n-D  NumberOfTableDimensions=1  BreakpointsForDimension1=spd_map_mot  Table=trq_map_mot  InternalRulePriority=Speed  RndMeth=Simplest  InputSameDT=on
  trq_dem_l : Outport
  trq_dem_r : Outport  Port=2
  trqlim_lf : Outport  Port=3
  trqlim_lr : Outport  Port=4
  trqlim_rf : Outport  Port=5
  trqlim_rr : Outport  Port=6
  wires:
  Gain2/1 -> Mux/2, Subtract/2, Add/2, Scope6/1
  Mux/1 -> Scope5/1
  MATLAB Function/2(trq_dem_r) -> trq_dem_r/1, Scope1/1
  MATLAB Function/1(trq_dem_l) -> trq_dem_l/1, Scope/1
  [delta_T_dem] -> MATLAB Function/5(delta_T_dem)
  [trqlim_r] -> Scope9/1, MinMax2/1, MATLAB Function/3(trqlim_r)
  Add2/1 -> [trqlim_r]
  [trqlim_l] -> MinMax1/1, MATLAB Function/1(trqlim_l), Scope4/1
  Add3/1 -> [trqlim_l]
  MinMax3/1 -> Add2/2, trqlim_rr/1
  MinMax4/1 -> Add2/1, trqlim_rf/1
  MinMax5/1 -> Add3/2, trqlim_lr/1
  MinMax6/1 -> Add3/1, trqlim_lf/1
  TrqLimU_dig_lf/1 -> MinMax6/2
  mot_map/1 -> MinMax6/1
  TrqLimU_dig_lr/1 -> MinMax5/2
  mot_map1/1 -> MinMax5/1
  TrqLimU_dig_rf/1 -> MinMax4/2
  mot_map2/1 -> MinMax4/1
  TrqLimU_dig_rr/1 -> MinMax3/2
  mot_map3/1 -> MinMax3/1
  MinMax2/1 -> MATLAB Function/4(trq_dem_r1), Scope7/1
  Add/1 -> MinMax2/2, Scope8/1
  MinMax1/1 -> MATLAB Function/2(trq_dem_l1), Scope3/1
  Subtract/1 -> MinMax1/2, Scope2/1
  delta_T_dem/1 -> Gain2/1, Scope10/1, [delta_T_dem]
  Gain1/1 -> Add/1, Subtract/1, Mux/1
  MinMax/1 -> Gain1/1
  Trq_line_dem/1 -> MinMax/2
  Divide/1 -> MinMax/1
  Gain/1 -> Divide/3
  pwr_dis_bat/1 -> Divide/2
  Constant/1 -> Divide/1
  Add1/1 -> Gain/1
  speed_act_lf/1 -> Add1/1, mot_map/1
  speed_act_rr/1 -> Add1/4, mot_map3/1
  speed_act_lr/1 -> Add1/2, mot_map1/1
  speed_act_rf/1 -> Add1/3, mot_map2/1

== system DDCU_wxt_v03/MainControl/mode_control/backward/backward/Drive/目标直驶力矩确定模块 ==
  acc_dem : Inport
  v_act : Inport  Port=2
  TrqLimU_dig_lf : Inport  Port=3
  TrqLimU_dig_lr : Inport  Port=4
  TrqLimU_dig_rf : Inport  Port=5
  TrqLimU_dig_rr : Inport  Port=6
  Add : Sum  Inputs=++++
  Constant : Constant  Value=3.6
  Constant1 : Constant  Value=Radius
  Constant2 : Constant  Value=30/pi
  Divide : Product  Inputs=*//*
  Gain : Gain  Gain=1/100
  Gain1 : Gain  Gain=tras_ratio
  MinMax{,1..3} (4 alike) : MinMax  Inputs=2
  Product : Product
  Scope : Scope
      settings: SaveName=ScopeData7
  Scope1 : Scope
      settings: SaveName=ScopeData8
  mot_map : Lookup_n-D  NumberOfTableDimensions=1  BreakpointsForDimension1=spd_map_mot  Table=trq_map_mot  InternalRulePriority=Speed  RndMeth=Simplest  InputSameDT=on
  Trq_line_dem : Outport
  wires:
  Gain1/1 -> mot_map/1
  Gain/1 -> Product/1
  Product/1 -> Trq_line_dem/1, Scope/1
  acc_dem/1 -> Gain/1
  Add/1 -> Product/2
  MinMax3/1 -> Add/4
  MinMax/1 -> Add/1
  MinMax2/1 -> Add/3
  MinMax1/1 -> Add/2
  TrqLimU_dig_rr/1 -> MinMax3/2
  TrqLimU_dig_rf/1 -> MinMax2/2
  TrqLimU_dig_lr/1 -> MinMax1/2
  mot_map/1 -> MinMax/1, Scope1/1, MinMax3/1, MinMax2/1, MinMax1/1
  TrqLimU_dig_lf/1 -> MinMax/2
  Divide/1 -> Gain1/1
  Constant2/1 -> Divide/4
  Constant/1 -> Divide/2
  Constant1/1 -> Divide/3
  v_act/1 -> Divide/1

== system DDCU_wxt_v03/MainControl/mode_control/backward/backward/Drive/目标转向力矩确定模块 ==
  note: 左转为正，右转为负
  v_act : Inport
  TrqLimU_dig_lf : Inport  Port=2
  TrqLimU_dig_lr : Inport  Port=3
  TrqLimU_dig_rf : Inport  Port=4
  TrqLimU_dig_rr : Inport  Port=5
  steer_dem : Inport  Port=6
  umax : Inport  Port=7
  f : Inport  Port=8
  Action Port : ActionPort
  Add : Sum
  Add1 : Sum
  Constant : Constant  Value=3.6
  Constant1 : Constant  Value=Radius
  Constant2 : Constant  Value=30/pi
  Constant3 : Constant  Value=G
  Constant4 : Constant  Value=L
  Constant5 : Constant  Value=B
  Constant6 : Constant  Value=eff_tran
  Constant7 : Constant  Value=Radius
  Constant8 : Constant  Value=ag_thr
  Constant9 : Constant  Value=Radius
  Divide : Product  Inputs=*//*
  Gain : Gain  Gain=1/100
  Gain1 : Gain  Gain=tras_ratio
  Gain2 : Gain  Gain=tras_ratio
  Gain3 : Gain  Gain=tras_ratio
  Gain4 : Gain  Gain=1/tras_ratio
  MATLAB Function : MATLAB Function  TreatAsAtomicUnit=on
  MATLAB Function1 : MATLAB Function  TreatAsAtomicUnit=on
  MATLAB Function2 : MATLAB Function  TreatAsAtomicUnit=on
  MinMax{,1..3} (4 alike) : MinMax  Inputs=2
  MinMax4 : MinMax  Function=max  Inputs=2
  Product : Product
  Scope{,1..3} (4 alike) : Scope
      Scope settings: SaveName=ScopeData10
      Scope1 settings: SaveName=ScopeData11
      Scope2 settings: SaveName=ScopeData12
      Scope3 settings: SaveName=ScopeData13
  mot_map : Lookup_n-D  NumberOfTableDimensions=1  BreakpointsForDimension1=spd_map_mot  Table=trq_map_mot  InternalRulePriority=Speed  RndMeth=Simplest  InputSameDT=on
  delta_Tsteer_dem : Outport
  wires:
  Gain1/1 -> mot_map/1
  MATLAB Function2/1(delta_Tsteer_max) -> Product/2, Scope2/1
  MinMax4/1 -> MATLAB Function2/6(Rturn_min_xy)
  Constant9/1 -> MATLAB Function2/5(Radius)
  [B] -> MATLAB Function2/4(B)
  [L] -> MATLAB Function2/3(L)
  [G] -> MATLAB Function2/2(G)
  [umax] -> MATLAB Function2/1(umax)
  MATLAB Function1/1(Rturn_min_ag) -> Scope1/1, MinMax4/2
  Constant8/1 -> MATLAB Function1/2(ag_thr)
  [v_act] -> MATLAB Function1/1(v_act)
  MATLAB Function/1(Rturn_min) -> MinMax4/1, Scope/1
  f/1 -> MATLAB Function/10(f)
  Constant7/1 -> MATLAB Function/9(Radius)
  Constant6/1 -> MATLAB Function/8(eff_tran)
  Add1/1 -> Gain3/1
  Add/1 -> Gain2/1
  umax/1 -> MATLAB Function/4(umax), [umax]
  Constant5/1 -> MATLAB Function/5(B), [B]
  Constant4/1 -> MATLAB Function/3(L), [L]
  Constant3/1 -> MATLAB Function/2(G), [G]
  steer_dem/1 -> MATLAB Function/1(steer_dem), [steer_dem]
  v_act/1 -> Divide/1, [v_act]
  Constant1/1 -> Divide/3
  Constant/1 -> Divide/2
  Constant2/1 -> Divide/4
  Divide/1 -> Gain1/1
  TrqLimU_dig_lf/1 -> MinMax/2
  mot_map/1 -> MinMax1/1, MinMax2/1, MinMax3/1, MinMax/1
  TrqLimU_dig_lr/1 -> MinMax1/2
  TrqLimU_dig_rf/1 -> MinMax2/2
  TrqLimU_dig_rr/1 -> MinMax3/2
  MinMax1/1 -> Add/2
  MinMax2/1 -> Add1/1
  MinMax/1 -> Add/1
  MinMax3/1 -> Add1/2
  [steer_dem] -> Gain/1
  Product/1 -> Gain4/1, Scope3/1
  Gain/1 -> Product/1
  Gain2/1 -> MATLAB Function/6(Tpeak_L)
  Gain3/1 -> MATLAB Function/7(Tpeak_R)
  Gain4/1 -> delta_Tsteer_dem/1

== system DDCU_wxt_v03/MainControl/mode_control/backward/backward/Drive/直驶纠偏控制 ==
  dis_east : Inport
  dis_north : Inport  Port=2
  hangxiangangle : Inport  Port=3
  Action Port : ActionPort
  Constant : Constant  Value=0
  Terminator : Terminator
  Terminator1 : Terminator
  Terminator2 : Terminator
  delta_Tjiupian : Outport
  wires:
  hangxiangangle/1 -> Terminator2/1
  dis_north/1 -> Terminator1/1
  dis_east/1 -> Terminator/1
  Constant/1 -> delta_Tjiupian/1

== system DDCU_wxt_v03/MainControl/mode_control/backward/backward/Drive/路面状况识别模块 ==
  In1 : Inport
  Constant : Constant  Value=0.9
  Constant1 : Constant  Value=0.05
  Constant2 : Constant  Value=0.15
  Constant3 : Constant  Value=0.15
  Terminator : Terminator
  umax : Outport
  f : Outport  Port=2
  s_opt_zhuan : Outport  Port=3
  s_opt_yi : Outport  Port=4
  wires:
  In1/1 -> Terminator/1
  Constant3/1 -> s_opt_yi/1
  Constant2/1 -> s_opt_zhuan/1
  Constant1/1 -> f/1
  Constant/1 -> umax/1

== system DDCU_wxt_v03/MainControl/mode_control/backward/backward/Drive/车辆稳定性控制 ==
  note: 加速度向左为正
  acc_y : Inport
  Action Port : ActionPort
  Abs : Abs
  Add : Sum  Inputs=+++
  Constant : Constant  Value=ag_thr
  Constant1 : Constant
  Constant2 : Constant  Value=-1
  Difference : simulink/Discrete/Difference  ICPrevInput=0.0  InputProcessing=Inherited  OutMin=[]  OutMax=[]  OutDataType=fixdt(1, 16)  OutScaling=2^-10  DoSatur=off
  Discrete-Time Integrator : DiscreteIntegrator  SampleTime=-1  ICPrevOutput=DiscIntNeverNeededParam  ICPrevScaledInput=DiscIntNeverNeededParam
  Gain : Gain  Gain=kp1
  Gain1 : Gain  Gain=ki1
  Gain2 : Gain  Gain=kd1
  Gain3 : Gain  Gain=1/tras_ratio
  Product : Product
  Sum : Sum  Inputs=|+-
  Switch : Switch
  delta_Twending_dem : Outport
  wires:
  Difference/1 -> Add/3
  Discrete-Time Integrator/1 -> Add/2
  Sum/1 -> Gain/1, Gain1/1, Gain2/1
  Add/1 -> Product/1
  Product/1 -> Gain3/1
  Switch/1 -> Product/2
  Constant2/1 -> Switch/3
  Constant1/1 -> Switch/1
  Abs/1 -> Sum/2
  Gain2/1 -> Difference/1
  Gain1/1 -> Discrete-Time Integrator/1
  Gain/1 -> Add/1
  acc_y/1 -> Abs/1, Switch/2
  Constant/1 -> Sum/1
  Gain3/1 -> delta_Twending_dem/1

== system DDCU_wxt_v03/MainControl/mode_control/backward/backward/Drive/驱动防滑控制TCS ==
  trq_dem_lf : Inport
  trq_dem_lr : Inport  Port=2
  trq_dem_rf : Inport  Port=3
  trq_dem_rr : Inport  Port=4
  bra_pre_l : Inport  Port=5
  bra_pre_r : Inport  Port=6
  speed_act_lf : Inport  Port=7
  speed_act_lr : Inport  Port=8
  speed_act_rf : Inport  Port=9
  speed_act_rr : Inport  Port=10
  v_act : Inport  Port=11
  steer_dem : Inport  Port=12
  acc_y : Inport  Port=13
  brake_dem : Inport  Port=14
  s_opt_zhuan : Inport  Port=15
  MATLAB Function : MATLAB Function  TreatAsAtomicUnit=on
  Multiport Switch : MultiPortSwitch  DataPortOrder=Zero-based contiguous  Inputs=2
  Switch Case : SwitchCase  CaseConditions={0,1}  ShowDefaultCase=off
  直行TCS : Subsystem  TreatAsAtomicUnit=on
  转向TCS : Subsystem  TreatAsAtomicUnit=on
  backward_dem : Outport
  wires:
  Multiport Switch/1 -> backward_dem/1
  转向TCS/1(backward_dem) -> Multiport Switch/2
  直行TCS/1(backward_dem) -> Multiport Switch/3
  brake_dem/1 -> 转向TCS/14(brake_dem), 直行TCS/14(brake_dem)
  s_opt_zhuan/1 -> 转向TCS/15(s_opt_zhuan), 直行TCS/15(s_opt_zhuan)
  acc_y/1 -> 转向TCS/13(acc_y), 直行TCS/13(acc_y)
  v_act/1 -> 转向TCS/12(v_act), 直行TCS/12(v_act)
  speed_act_rr/1 -> 转向TCS/11(speed_act_rr), 直行TCS/11(speed_act_rr)
  speed_act_rf/1 -> 转向TCS/10(speed_act_rf), 直行TCS/10(speed_act_rf)
  speed_act_lr/1 -> 转向TCS/9(speed_act_lr), 直行TCS/9(speed_act_lr)
  speed_act_lf/1 -> 转向TCS/8(speed_act_lf), 直行TCS/8(speed_act_lf)
  bra_pre_r/1 -> 转向TCS/7(bra_pre_r), 直行TCS/7(bra_pre_r)
  bra_pre_l/1 -> 转向TCS/6(bra_pre_l), 直行TCS/6(bra_pre_l)
  trq_dem_rr/1 -> 转向TCS/5(trq_dem_rr), 直行TCS/5(trq_dem_rr)
  trq_dem_rf/1 -> 转向TCS/4(trq_dem_rf), 直行TCS/4(trq_dem_rf)
  trq_dem_lr/1 -> 转向TCS/3(trq_dem_lr), 直行TCS/3(trq_dem_lr)
  trq_dem_lf/1 -> 转向TCS/2(trq_dem_lf), 直行TCS/2(trq_dem_lf)
  Switch Case/2 -> 直行TCS/Action
  Switch Case/1 -> 转向TCS/Action
  MATLAB Function/1(y) -> Switch Case/1, Multiport Switch/1
  steer_dem/1 -> MATLAB Function/1(steer_dem), 直行TCS/1(steer_dem), 转向TCS/1(steer_dem)

== system DDCU_wxt_v03/MainControl/mode_control/forward/forward/Brake/Subsystem ==
  s_opt_yi : Inport
  syi_act_lf : Inport  Port=2
  syi_act_lr : Inport  Port=3
  syi_act_rf : Inport  Port=4
  syi_act_rr : Inport  Port=5
  flagyi_lf : Inport  Port=6
  flagyi_lr : Inport  Port=7
  flagyi_rf : Inport  Port=8
  flagyi_rr : Inport  Port=9
  bratrq_dem_lf : Inport  Port=10
  bratrq_dem_lr : Inport  Port=11
  bratrq_dem_rf : Inport  Port=12
  bratrq_dem_rr : Inport  Port=13
  Add{1..2,5,7} (4 alike) : Sum  Inputs=+++
  Add{3..4,6,8} (4 alike) : Sum
  Difference{,1..3} (4 alike) : simulink/Discrete/Difference  ICPrevInput=0.0  InputProcessing=Inherited  OutMin=[]  OutMax=[]  OutDataType=fixdt(1, 16)  OutScaling=2^-10  DoSatur=off
  Discrete-Time Integrator{,1..3} (4 alike) : DiscreteIntegrator  SampleTime=-1  ICPrevOutput=DiscIntNeverNeededParam  ICPrevScaledInput=DiscIntNeverNeededParam
  Gain{1,4,7,10} (4 alike) : Gain  Gain=kp3
  Gain{2,5,8,11} (4 alike) : Gain  Gain=ki3
  Gain{3,6,9,12} (4 alike) : Gain  Gain=kd3
  Sum{,1..3} (4 alike) : Sum  Inputs=|+-
  Switch{,1..3} (4 alike) : Switch  Criteria=u2 > Threshold  Threshold=0.5
  bratrq_pid_lf : Outport
  bratrq_pid_lr : Outport  Port=2
  bratrq_pid_rf : Outport  Port=3
  bratrq_pid_rr : Outport  Port=4
  wires:
  Add3/1 -> Switch/1
  bratrq_dem_lf/1 -> Switch/3, Add3/2
  syi_act_lf/1 -> Sum/2
  Difference/1 -> Add2/3
  Discrete-Time Integrator/1 -> Add2/2
  Gain3/1 -> Difference/1
  Gain1/1 -> Add2/1
  Gain2/1 -> Discrete-Time Integrator/1
  s_opt_yi/1 -> [s_opt_yi], Sum/1
  flagyi_lf/1 -> Switch/2
  Switch/1 -> bratrq_pid_lf/1
  Add4/1 -> Switch1/1
  bratrq_dem_lr/1 -> Switch1/3, Add4/2
  syi_act_lr/1 -> Sum1/2
  Difference1/1 -> Add1/3
  Discrete-Time Integrator1/1 -> Add1/2
  Gain6/1 -> Difference1/1
  Gain4/1 -> Add1/1
  Gain5/1 -> Discrete-Time Integrator1/1
  [s_opt_yi] -> Sum1/1
  flagyi_lr/1 -> Switch1/2
  Switch1/1 -> bratrq_pid_lr/1
  Add6/1 -> Switch2/1
  bratrq_dem_rr/1 -> Switch2/3, Add6/2
  syi_act_rr/1 -> Sum2/2
  Difference2/1 -> Add5/3
  Discrete-Time Integrator2/1 -> Add5/2
  Gain9/1 -> Difference2/1
  Gain7/1 -> Add5/1
  Gain8/1 -> Discrete-Time Integrator2/1
  [s_opt_yi] -> Sum2/1
  flagyi_rr/1 -> Switch2/2
  Switch2/1 -> bratrq_pid_rr/1
  Add8/1 -> Switch3/1
  bratrq_dem_rf/1 -> Switch3/3, Add8/2
  syi_act_rf/1 -> Sum3/2
  Difference3/1 -> Add7/3
  Discrete-Time Integrator3/1 -> Add7/2
  Gain12/1 -> Difference3/1
  Gain10/1 -> Add7/1
  Gain11/1 -> Discrete-Time Integrator3/1
  [s_opt_yi] -> Sum3/1
  flagyi_rf/1 -> Switch3/2
  Switch3/1 -> bratrq_pid_rf/1
  Add2/1 -> Add3/1
  Sum/1 -> Gain2/1, Gain3/1, Gain1/1
  Add1/1 -> Add4/1
  Sum1/1 -> Gain6/1, Gain5/1, Gain4/1
  Add7/1 -> Add8/1
  Sum3/1 -> Gain11/1, Gain12/1, Gain10/1
  Add5/1 -> Add6/1
  Sum2/1 -> Gain8/1, Gain9/1, Gain7/1

== system DDCU_wxt_v03/MainControl/mode_control/forward/forward/Brake/Subsystem1 ==
  speed_act_lf : Inport
  speed_act_lr : Inport  Port=2
  speed_act_rf : Inport  Port=3
  speed_act_rr : Inport  Port=4
  mot_map{,1..3} (4 alike) : Lookup_n-D  NumberOfTableDimensions=1  BreakpointsForDimension1=spd_map_mot  Table=trq_map_mot  InternalRulePriority=Speed  RndMeth=Simplest  InputSameDT=on
  trqlim_map_lf : Outport
  trqlim_map_lr : Outport  Port=2
  trqlim_map_rf : Outport  Port=3
  trqlim_map_rr : Outport  Port=4
  wires:
  speed_act_lf/1 -> mot_map/1
  speed_act_lr/1 -> mot_map1/1
  speed_act_rf/1 -> mot_map2/1
  speed_act_rr/1 -> mot_map3/1
  mot_map/1 -> trqlim_map_lf/1
  mot_map1/1 -> trqlim_map_lr/1
  mot_map2/1 -> trqlim_map_rf/1
  mot_map3/1 -> trqlim_map_rr/1

== system DDCU_wxt_v03/MainControl/mode_control/forward/forward/Brake/lf ==
  speed_act_lf : Inport
  v_act : Inport  Port=2
  Add : Sum
  Constant : Constant  Value=eps
  Divide : Product  Inputs=*/
  Gain : Gain  Gain=pi/30
  Gain1 : Gain  Gain=Radius
  Gain2 : Gain  Gain=1/3.6
  Subtract : Sum  Inputs=+-
  syi_act_lf : Outport
  wires:
  Divide/1 -> syi_act_lf/1
  Add/1 -> Divide/2
  Constant/1 -> Add/2
  Subtract/1 -> Divide/1
  v_act/1 -> Gain2/1
  Gain/1 -> Gain1/1
  speed_act_lf/1 -> Gain/1
  Gain2/1 -> Add/1, Subtract/1
  Gain1/1 -> Subtract/2

== system DDCU_wxt_v03/MainControl/mode_control/forward/forward/Brake/lr ==
  speed_act_lr : Inport
  v_act : Inport  Port=2
  Add : Sum
  Constant : Constant  Value=eps
  Divide : Product  Inputs=*/
  Gain : Gain  Gain=pi/30
  Gain1 : Gain  Gain=Radius
  Gain2 : Gain  Gain=1/3.6
  Subtract : Sum  Inputs=+-
  syi_act_lr : Outport
  wires:
  speed_act_lr/1 -> Gain/1
  Gain/1 -> Gain1/1
  v_act/1 -> Gain2/1
  Subtract/1 -> Divide/1
  Constant/1 -> Add/2
  Add/1 -> Divide/2
  Divide/1 -> syi_act_lr/1
  Gain1/1 -> Subtract/2
  Gain2/1 -> Add/1, Subtract/1

== system DDCU_wxt_v03/MainControl/mode_control/forward/forward/Brake/rf ==
  speed_act_rf : Inport
  v_act : Inport  Port=2
  Add : Sum
  Constant : Constant  Value=eps
  Divide : Product  Inputs=*/
  Gain : Gain  Gain=pi/30
  Gain1 : Gain  Gain=Radius
  Gain2 : Gain  Gain=1/3.6
  Subtract : Sum  Inputs=+-
  syi_act_rf : Outport
  wires:
  Divide/1 -> syi_act_rf/1
  Add/1 -> Divide/2
  Constant/1 -> Add/2
  Subtract/1 -> Divide/1
  v_act/1 -> Gain2/1
  Gain/1 -> Gain1/1
  speed_act_rf/1 -> Gain/1
  Gain2/1 -> Add/1, Subtract/1
  Gain1/1 -> Subtract/2

== system DDCU_wxt_v03/MainControl/mode_control/forward/forward/Brake/rr ==
  speed_act_rr : Inport
  v_act : Inport  Port=2
  Add : Sum
  Constant : Constant  Value=eps
  Divide : Product  Inputs=*/
  Gain : Gain  Gain=pi/30
  Gain1 : Gain  Gain=Radius
  Gain2 : Gain  Gain=1/3.6
  Subtract : Sum  Inputs=+-
  s_act_rr : Outport
  wires:
  speed_act_rr/1 -> Gain/1
  Gain/1 -> Gain1/1
  v_act/1 -> Gain2/1
  Subtract/1 -> Divide/1
  Constant/1 -> Add/2
  Add/1 -> Divide/2
  Divide/1 -> s_act_rr/1
  Gain2/1 -> Add/1, Subtract/1
  Gain1/1 -> Subtract/2

== system DDCU_wxt_v03/MainControl/mode_control/forward/forward/Drive/容错控制 ==
  trq_dem_l : Inport
  trq_dem_r : Inport  Port=2
  trqlim_lf : Inport  Port=3
  trqlim_lr : Inport  Port=4
  trqlim_rf : Inport  Port=5
  trqlim_rr : Inport  Port=6
  guzhang_lf : Inport  Port=7
  guzhang_lr : Inport  Port=8
  guzhang_rf : Inport  Port=9
  guzhang_rr : Inport  Port=10
  Add : Sum
  Add1 : Sum
  Constant : Constant  Value=bra_pre_gz2
  Constant1 : Constant  Value=bra_pre_gz34
  MATLAB Function : MATLAB Function  TreatAsAtomicUnit=on
  Mux : Mux  Inputs=2
  Scope{,1..16} (17 alike) : Scope
      Scope settings: SaveName=ScopeData25
      Scope1 settings: SaveName=ScopeData26
      Scope10 settings: SaveName=ScopeData35
      Scope11 settings: SaveName=ScopeData36
      Scope12 settings: SaveName=ScopeData37
      Scope13 settings: SaveName=ScopeData38
      Scope14 settings: SaveName=ScopeData39
      Scope15 settings: SaveName=ScopeData40
      Scope16 settings: SaveName=ScopeData41
      Scope2 settings: SaveName=ScopeData27
      Scope3 settings: SaveName=ScopeData28
      Scope4 settings: SaveName=ScopeData29
      Scope5 settings: SaveName=ScopeData30
      Scope6 settings: SaveName=ScopeData31
      Scope7 settings: SaveName=ScopeData32
      Scope8 settings: SaveName=ScopeData33
      Scope9 settings: SaveName=ScopeData34
  Subtract : Sum  Inputs=+-
  To Workspace1 : ToWorkspace  VariableName=simout1  SaveFormat=Timeseries  SampleTime=-1
  To Workspace2 : ToWorkspace  VariableName=simout  SaveFormat=Timeseries  SampleTime=-1
  To Workspace3 : ToWorkspace  VariableName=simout2  SaveFormat=Timeseries  SampleTime=-1
  To Workspace4 : ToWorkspace  VariableName=simout3  SaveFormat=Timeseries  SampleTime=-1
  To Workspace5 : ToWorkspace  VariableName=simout4  SaveFormat=Timeseries  SampleTime=-1
  trq_dem_lf : Outport
  trq_dem_lr : Outport  Port=2
  trq_dem_rf : Outport  Port=3
  trq_dem_rr : Outport  Port=4
  bra_pre_l : Outport  Port=5
  bra_pre_r : Outport  Port=6
  wires:
  guzhang_lr/1 -> To Workspace3/1, MATLAB Function/8(guzhang_lr), Scope14/1
  guzhang_rf/1 -> Scope15/1, To Workspace4/1, MATLAB Function/9(guzhang_rf)
  guzhang_rr/1 -> Scope16/1, To Workspace5/1, MATLAB Function/10(guzhang_rr)
  guzhang_lf/1 -> To Workspace2/1, Scope13/1, MATLAB Function/7(guzhang_lf)
  trq_dem_r/1 -> Scope9/1, MATLAB Function/2(trq_dem_r)
  trqlim_lr/1 -> MATLAB Function/4(trqlim_lr)
  trq_dem_l/1 -> Scope8/1, MATLAB Function/1(trq_dem_l)
  trqlim_rf/1 -> Scope10/1, MATLAB Function/5(trqlim_rf)
  trqlim_rr/1 -> Scope12/1, MATLAB Function/6(trqlim_rr)
  trqlim_lf/1 -> MATLAB Function/3(trqlim_lf)
  MATLAB Function/1(trq_dem_lf) -> Scope/1, Add/1, trq_dem_lf/1
  MATLAB Function/2(trq_dem_lr) -> Scope1/1, Add/2, trq_dem_lr/1
  MATLAB Function/3(trq_dem_rf) -> Scope2/1, Add1/1, trq_dem_rf/1
  MATLAB Function/4(trq_dem_rr) -> Scope3/1, Add1/2, trq_dem_rr/1
  MATLAB Function/5(bra_pre_l) -> Scope4/1, bra_pre_l/1
  MATLAB Function/6(bra_pre_r) -> Scope5/1, bra_pre_r/1
  Constant/1 -> MATLAB Function/11(bra_pre_gz2)
  Constant1/1 -> MATLAB Function/12(bra_pre_gz34)
  Add/1 -> Mux/1, Subtract/1
  Add1/1 -> Mux/2, Subtract/2
  Subtract/1 -> Scope6/1
  Mux/1 -> Scope7/1
  MATLAB Function/7(mode) -> To Workspace1/1, Scope11/1
